simulink model "stepping_control"  (Simulink 3.00)
settings: Solver=FixedStepDiscrete  StartTime=0.0  StopTime=500.0  FixedStep=0.1  RelTol=1e-3
libraries: mathlib x5, genlib x2, reglib x2, arclib x2, execlib x1
settings Model: LastModifiedBy=mertlj

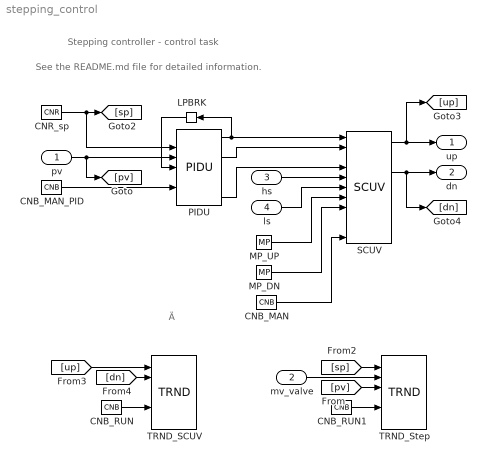
== system stepping_control ==
  note: Ä
  note: See the README.md file for detailed information.
  note: Stepping controller - control task
  pv : Inport  Port=1
  mv_valve : Inport  Port=2
  hs : Inport  Port=3
  ls : Inport  Port=4
  CNB_MAN : mathlib/CNB  YCN=off
  CNB_MAN_PID : mathlib/CNB  YCN=off
  CNB_RUN : mathlib/CNB  YCN=on
  CNB_RUN1 : mathlib/CNB  YCN=on
  CNR_sp : mathlib/CNR  ycn=0
  LPBRK : execlib/LPBRK  Orientation=left
  MP_DN : genlib/MP  pwidth=1  BSTATE=off  RPTF=off
  MP_UP : genlib/MP  pwidth=1  BSTATE=off  RPTF=off
  PIDU : reglib/PIDU  irtype=7: PID  RACT=off  k=1.8  ti=21  td=4.3  nd=2  b=1  c=0  tt=1  hilim=1  lolim=0  dz=0  icotype=4: SCUV
  SCUV : reglib/SCUV  thron=0.002  throff=0.001  dtime=0.01  btime=0.01  RACT=off  trun=10  CWOI=off  tt=1
  TRND_SCUV : arclib/TRND  n=2  l=1000  btype=8  ptype1=1: Store  ptype2=1: Store  ptype3=1: Store  ptype4=1: Store  pfac=1  afac=0  arc=0  id=1  Title=Trend Title  timesrc=1
  TRND_Step : arclib/TRND  n=3  l=1000  btype=8  ptype1=1: Store  ptype2=1: Store  ptype3=1: Store  ptype4=1: Store  pfac=1  afac=0  arc=0  id=2  Title=Trend Title  timesrc=1
  up : Outport  Port=1
  dn : Outport  Port=2
  wires:
  CNB_MAN/1 -> SCUV/11
  CNB_MAN_PID/1 -> PIDU/6
  CNB_RUN/1 -> TRND_SCUV/5
  CNB_RUN1/1 -> TRND_Step/5
  CNR_sp/1 -> [sp], PIDU/2
  [pv] -> TRND_Step/3
  [sp] -> TRND_Step/1
  [up] -> TRND_SCUV/1
  [dn] -> TRND_SCUV/2
  LPBRK/1 -> PIDU/4
  MP_DN/1 -> SCUV/8
  MP_UP/1 -> SCUV/7
  PIDU/1 -> LPBRK/1, SCUV/1
  PIDU/2 -> SCUV/2
  PIDU/4 -> SCUV/4
  SCUV/1 -> [up], up/1
  SCUV/2 -> [dn], dn/1
  hs/1 -> SCUV/5
  ls/1 -> SCUV/6
  mv_valve/1 -> TRND_Step/2
  pv/1 -> [pv], PIDU/3
